simulink subsystem "SiMappedEngine"  (R2025a)
settings: Solver=VariableStepAuto  StartTime=0.0  StopTime=10.0  RelTol=1e-3
undefined symbols (not defined in the file): Afr, BSFC, Ect, EgrVlvAreaPct, EngSpdOut, EngTrq, ExhCamPhase, ExhManGasTemp, FuelFlw, FuelVolFlw, IntkCamPhase, IntkPortFlw, IntkSwirlVlvPos, IntkVlvLift, NormAirChrg, PlntEngAfrStoich, PlntEngTimeCECP, PlntEngTimeCEGR, PlntEngTimeCETC, PlntEngTimeCICP, PlntEngTimeCIRL, PlntEngTimeCIVL, PlntEngTimeCVCR, PlntEngTimeCVGT, PlntEngTimeCWGA, PlntEngTimeCWVA, PlntEngTwcEffCO, PlntEngTwcEffHC, PlntEngTwcEffLam, PlntEngTwcEffNOx, ThrPosPct, TPCO, TPCO2, TPHC, TPNOx, TurboRackPos, VarCompRatioPos, VarIntkRunLen, WgAreaPct
libraries: autolibsharedcommon x1, autolibpowerinfoutils x1, autolibsharedmappedengines x1, autolibutils x1
(part 2 of 2)

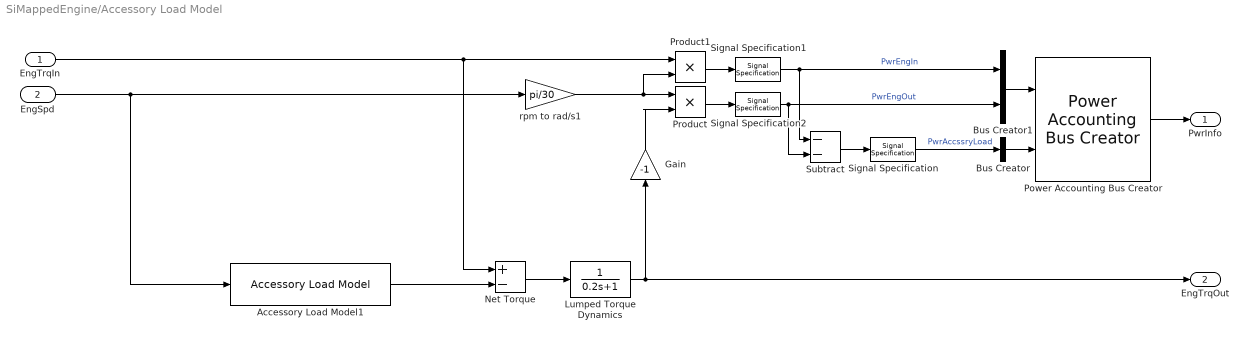
== system SiMappedEngine/Accessory Load Model ==
  EngTrqIn : Inport
  EngSpd : Inport  Port=2
  Accessory Load Model1 : autolibsharedcommon/Accessory Load Model  AccPwrTbl=PlntEngAccPwrTbl  AccSpdBpts=PlntEngAccSpdBpt  aMode=aMode
  Bus Creator : BusCreator  Inputs=1
  Bus Creator1 : BusCreator  Inputs=2
  Gain : Gain  Gain=-1
  Lumped Torque Dynamics : TransferFcn  Denominator=[0.2 1]
  Net Torque : Sum  Inputs=+-
  Power Accounting Bus Creator : autolibpowerinfoutils/Power Accounting Bus Creator  AssctBlkSelPopup=Parent  RefBlkName='libraryname/blkname'  PwrTrnsfrdCheckBox=on  PwrNotTrnsfrdCheckBox=on  PwrStoredCheckBox=off  aMode=6
  Product : Product
  Product1 : Product
  Signal Specification : SignalSpecification  Unit=W
  Signal Specification1 : SignalSpecification  Unit=W
  Signal Specification2 : SignalSpecification  Unit=W
  Subtract : Sum  Inputs=--
  rpm to rad/s1 : Gain  Gain=pi/30
  PwrInfo : Outport  VectorParamsAs1DForOutWhenUnconnected=off
  EngTrqOut : Outport  Port=2  Unit=N*m  VectorParamsAs1DForOutWhenUnconnected=off
  wires:
  Gain/1 -> Product/2
  Signal Specification2/1 -> Bus Creator1/2, Subtract/2  "PwrEngOut"
  Signal Specification1/1 -> Bus Creator1/1, Subtract/1  "PwrEngIn"
  rpm to rad/s1/1 -> Product/1, Product1/2
  Product1/1 -> Signal Specification1/1
  Product/1 -> Signal Specification2/1
  Power Accounting Bus Creator/1 -> PwrInfo/1
  Signal Specification/1 -> Bus Creator/1  "PwrAccssryLoad"
  Subtract/1 -> Signal Specification/1
  EngTrqIn/1 -> Net Torque/1, Product1/1
  Bus Creator1/1 -> Power Accounting Bus Creator/1
  Bus Creator/1 -> Power Accounting Bus Creator/2
  Net Torque/1 -> Lumped Torque Dynamics/1
  Lumped Torque Dynamics/1 -> Gain/1, EngTrqOut/1
  EngSpd/1 -> Accessory Load Model1/1, rpm to rad/s1/1
  Accessory Load Model1/1 -> Net Torque/2

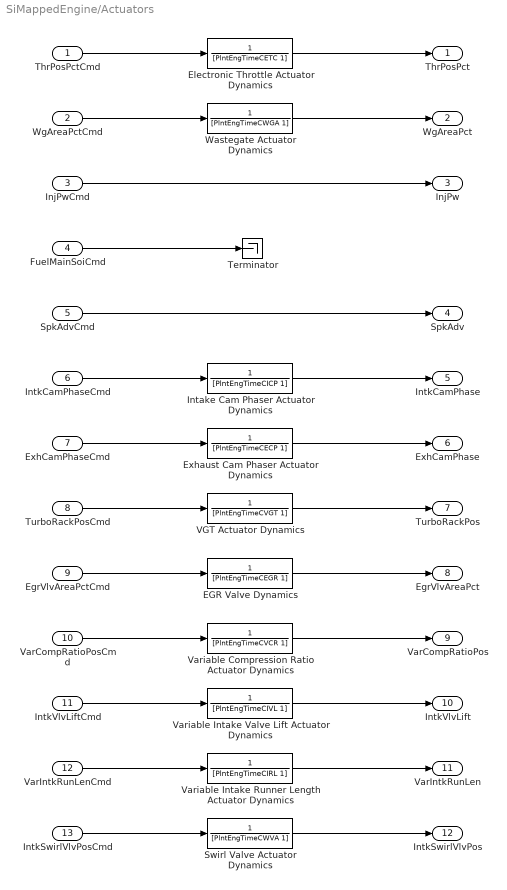
== system SiMappedEngine/Actuators ==
  ThrPosPctCmd : Inport  Unit=%
  WgAreaPctCmd : Inport  Port=2  Unit=%
  InjPwCmd : Inport  Port=3  Unit=ms
  FuelMainSoiCmd : Inport  Port=4  Unit=deg
  SpkAdvCmd : Inport  Port=5  Unit=deg
  IntkCamPhaseCmd : Inport  Port=6  Unit=deg
  ExhCamPhaseCmd : Inport  Port=7  Unit=deg
  TurboRackPosCmd : Inport  Port=8  Unit=1
  EgrVlvAreaPctCmd : Inport  Port=9  Unit=%
  VarCompRatioPosCmd : Inport  Port=10
  IntkVlvLiftCmd : Inport  Port=11
  VarIntkRunLenCmd : Inport  Port=12
  IntkSwirlVlvPosCmd : Inport  Port=13
  EGR Valve Dynamics : TransferFcn  Denominator=[PlntEngTimeCEGR 1]
  Electronic Throttle Actuator Dynamics : TransferFcn  Denominator=[PlntEngTimeCETC 1]
  Exhaust Cam Phaser Actuator Dynamics : TransferFcn  Denominator=[PlntEngTimeCECP 1]
  Intake Cam Phaser Actuator Dynamics : TransferFcn  Denominator=[PlntEngTimeCICP 1]
  Swirl Valve Actuator Dynamics : TransferFcn  Denominator=[PlntEngTimeCWVA 1]
  Terminator : Terminator
  VGT Actuator Dynamics : TransferFcn  Denominator=[PlntEngTimeCVGT 1]
  Variable Compression Ratio Actuator Dynamics : TransferFcn  Denominator=[PlntEngTimeCVCR 1]
  Variable Intake Runner Length Actuator Dynamics : TransferFcn  Denominator=[PlntEngTimeCIRL 1]
  Variable Intake Valve Lift Actuator Dynamics : TransferFcn  Denominator=[PlntEngTimeCIVL 1]
  Wastegate Actuator Dynamics : TransferFcn  Denominator=[PlntEngTimeCWGA 1]
  ThrPosPct : Outport  Unit=%  VectorParamsAs1DForOutWhenUnconnected=off
  WgAreaPct : Outport  Port=2  Unit=%  VectorParamsAs1DForOutWhenUnconnected=off
  InjPw : Outport  Port=3  VectorParamsAs1DForOutWhenUnconnected=off
  SpkAdv : Outport  Port=4  VectorParamsAs1DForOutWhenUnconnected=off
  IntkCamPhase : Outport  Port=5  Unit=deg  VectorParamsAs1DForOutWhenUnconnected=off
  ExhCamPhase : Outport  Port=6  Unit=deg  VectorParamsAs1DForOutWhenUnconnected=off
  TurboRackPos : Outport  Port=7  Unit=1  VectorParamsAs1DForOutWhenUnconnected=off
  EgrVlvAreaPct : Outport  Port=8  Unit=%  VectorParamsAs1DForOutWhenUnconnected=off
  VarCompRatioPos : Outport  Port=9  VectorParamsAs1DForOutWhenUnconnected=off
  IntkVlvLift : Outport  Port=10  VectorParamsAs1DForOutWhenUnconnected=off
  VarIntkRunLen : Outport  Port=11  VectorParamsAs1DForOutWhenUnconnected=off
  IntkSwirlVlvPos : Outport  Port=12  VectorParamsAs1DForOutWhenUnconnected=off
  wires:
  SpkAdvCmd/1 -> SpkAdv/1
  EgrVlvAreaPctCmd/1 -> EGR Valve Dynamics/1
  TurboRackPosCmd/1 -> VGT Actuator Dynamics/1
  EGR Valve Dynamics/1 -> EgrVlvAreaPct/1
  VGT Actuator Dynamics/1 -> TurboRackPos/1
  InjPwCmd/1 -> InjPw/1
  VarIntkRunLenCmd/1 -> Variable Intake Runner Length Actuator Dynamics/1
  VarCompRatioPosCmd/1 -> Variable Compression Ratio Actuator Dynamics/1
  IntkCamPhaseCmd/1 -> Intake Cam Phaser Actuator Dynamics/1
  ExhCamPhaseCmd/1 -> Exhaust Cam Phaser Actuator Dynamics/1
  ThrPosPctCmd/1 -> Electronic Throttle Actuator Dynamics/1
  WgAreaPctCmd/1 -> Wastegate Actuator Dynamics/1
  IntkSwirlVlvPosCmd/1 -> Swirl Valve Actuator Dynamics/1
  IntkVlvLiftCmd/1 -> Variable Intake Valve Lift Actuator Dynamics/1
  FuelMainSoiCmd/1 -> Terminator/1
  Electronic Throttle Actuator Dynamics/1 -> ThrPosPct/1
  Wastegate Actuator Dynamics/1 -> WgAreaPct/1
  Exhaust Cam Phaser Actuator Dynamics/1 -> ExhCamPhase/1
  Intake Cam Phaser Actuator Dynamics/1 -> IntkCamPhase/1
  Swirl Valve Actuator Dynamics/1 -> IntkSwirlVlvPos/1
  Variable Intake Runner Length Actuator Dynamics/1 -> VarIntkRunLen/1
  Variable Intake Valve Lift Actuator Dynamics/1 -> IntkVlvLift/1
  Variable Compression Ratio Actuator Dynamics/1 -> VarCompRatioPos/1

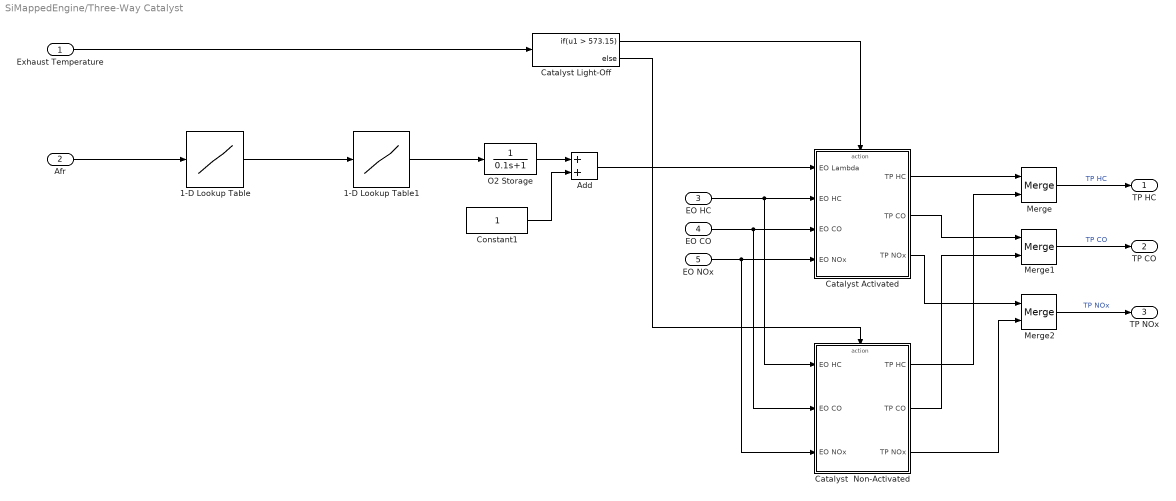
== system SiMappedEngine/Three-Way Catalyst ==
  Exhaust Temperature : Inport
  Afr : Inport  Port=2
  EO HC : Inport  Port=3
  EO CO : Inport  Port=4
  EO NOx : Inport  Port=5
  1-D Lookup Table : Lookup_n-D  NumberOfTableDimensions=1  BreakpointsForDimension1=[0 15 100]  Table=[0 15 PlntEngAfrStoich]/PlntEngAfrStoich  ExtrapMethod=Clip  InternalRulePriority=Speed  RndMeth=Simplest
  1-D Lookup Table1 : Lookup_n-D  NumberOfTableDimensions=1  BreakpointsForDimension1=[0 0.97 1.03 1.1]  Table=[-1 0 0 0.07]  ExtrapMethod=Clip  InternalRulePriority=Speed  RndMeth=Simplest
  Add : Sum
  Catalyst  Non-Activated : Subsystem
  Catalyst Activated : Subsystem
  Catalyst Light-Off : If  IfExpression=u1 > 573.15
  Constant1 : Constant
  Merge : Merge
  Merge1 : Merge
  Merge2 : Merge
  O2 Storage : TransferFcn  Denominator=[0.1 1]
  TP HC : Outport  Unit=kg/s  VectorParamsAs1DForOutWhenUnconnected=off
  TP CO : Outport  Port=2  Unit=kg/s  VectorParamsAs1DForOutWhenUnconnected=off
  TP NOx : Outport  Port=3  Unit=kg/s  VectorParamsAs1DForOutWhenUnconnected=off
  wires:
  Afr/1 -> 1-D Lookup Table/1
  1-D Lookup Table/1 -> 1-D Lookup Table1/1
  Add/1 -> Catalyst Activated/1(EO Lambda)
  O2 Storage/1 -> Add/1
  Constant1/1 -> Add/2
  1-D Lookup Table1/1 -> O2 Storage/1
  Catalyst  Non-Activated/3(TP NOx) -> Merge2/2
  Catalyst Activated/3(TP NOx) -> Merge2/1
  Catalyst  Non-Activated/2(TP CO) -> Merge1/2
  Catalyst Activated/2(TP CO) -> Merge1/1
  Catalyst  Non-Activated/1(TP HC) -> Merge/2
  Catalyst Activated/1(TP HC) -> Merge/1
  Exhaust Temperature/1 -> Catalyst Light-Off/1
  Catalyst Light-Off/2 -> Catalyst  Non-Activated/Action
  Catalyst Light-Off/1 -> Catalyst Activated/Action
  Merge2/1 -> TP NOx/1  "TP NOx"
  Merge1/1 -> TP CO/1  "TP CO"
  Merge/1 -> TP HC/1  "TP HC"
  EO NOx/1 -> Catalyst Activated/4(EO NOx), Catalyst  Non-Activated/3(EO NOx)
  EO CO/1 -> Catalyst Activated/3(EO CO), Catalyst  Non-Activated/2(EO CO)
  EO HC/1 -> Catalyst Activated/2(EO HC), Catalyst  Non-Activated/1(EO HC)

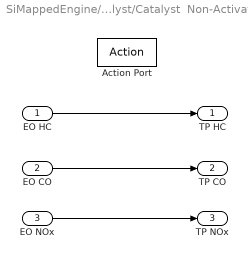
== system SiMappedEngine/Three-Way Catalyst/Catalyst  Non-Activated ==
  EO HC : Inport
  EO CO : Inport  Port=2
  EO NOx : Inport  Port=3
  Action Port : ActionPort
  TP HC : Outport  VectorParamsAs1DForOutWhenUnconnected=off
  TP CO : Outport  Port=2  VectorParamsAs1DForOutWhenUnconnected=off
  TP NOx : Outport  Port=3  VectorParamsAs1DForOutWhenUnconnected=off
  wires:
  EO NOx/1 -> TP NOx/1
  EO CO/1 -> TP CO/1
  EO HC/1 -> TP HC/1

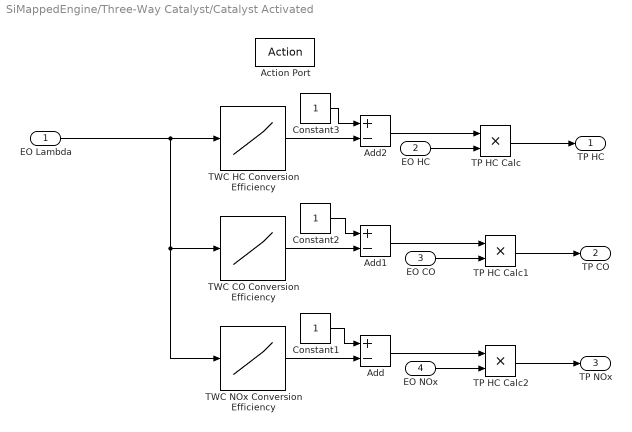
== system SiMappedEngine/Three-Way Catalyst/Catalyst Activated ==
  EO Lambda : Inport
  EO HC : Inport  Port=2
  EO CO : Inport  Port=3
  EO NOx : Inport  Port=4
  Action Port : ActionPort
  Add : Sum  Inputs=+-
  Add1 : Sum  Inputs=+-
  Add2 : Sum  Inputs=+-
  Constant1 : Constant
  Constant2 : Constant
  Constant3 : Constant
  TP HC Calc : Product  Inputs=**
  TP HC Calc1 : Product  Inputs=**
  TP HC Calc2 : Product  Inputs=**
  TWC CO Conversion Efficiency : Lookup_n-D  NumberOfTableDimensions=1  LookupTableObject=''  BreakpointsForDimension1=PlntEngTwcEffLam  Table=PlntEngTwcEffCO  ExtrapMethod=Clip  InternalRulePriority=Speed  RndMeth=Simplest
  TWC HC Conversion Efficiency : Lookup_n-D  NumberOfTableDimensions=1  LookupTableObject=''  BreakpointsForDimension1=PlntEngTwcEffLam  Table=PlntEngTwcEffHC  ExtrapMethod=Clip  InternalRulePriority=Speed  RndMeth=Simplest
  TWC NOx Conversion Efficiency : Lookup_n-D  NumberOfTableDimensions=1  LookupTableObject=''  BreakpointsForDimension1=PlntEngTwcEffLam  Table=PlntEngTwcEffNOx  ExtrapMethod=Clip  InternalRulePriority=Speed  RndMeth=Simplest
  TP HC : Outport  VectorParamsAs1DForOutWhenUnconnected=off
  TP CO : Outport  Port=2  VectorParamsAs1DForOutWhenUnconnected=off
  TP NOx : Outport  Port=3  VectorParamsAs1DForOutWhenUnconnected=off
  wires:
  Add2/1 -> TP HC Calc/1
  Constant3/1 -> Add2/1
  TWC CO Conversion Efficiency/1 -> Add1/2
  Constant2/1 -> Add1/1
  EO Lambda/1 -> TWC HC Conversion Efficiency/1, TWC CO Conversion Efficiency/1, TWC NOx Conversion Efficiency/1
  EO NOx/1 -> TP HC Calc2/2
  TP HC Calc2/1 -> TP NOx/1
  TWC NOx Conversion Efficiency/1 -> Add/2
  EO CO/1 -> TP HC Calc1/2
  Add1/1 -> TP HC Calc1/1
  TWC HC Conversion Efficiency/1 -> Add2/2
  TP HC Calc1/1 -> TP CO/1
  Constant1/1 -> Add/1
  Add/1 -> TP HC Calc2/1
  TP HC Calc/1 -> TP HC/1
  EO HC/1 -> TP HC Calc/2
